simulink model "drone"  (Simulink 6.1)
settings: Solver=ode5  StartTime=0.0  StopTime=90  FixedStep=1e-2  RelTol=1e-3
undefined symbols (not defined in the file or in its folder): Aerodynamique, Correcteur, Mecanique
libraries: simulink x32, mblibv1 x29, aerolibtransform2 x4
(part 2 of 2)

== system drone/Electronique/Gestion Dynamique/Calcul Attitude/Norme ==
  Entrée : Inport  Port=1  LatchInput=off
  Add : Sum  Inputs=+++  OutScaling=2^-10
  Carré : simulink/Math Operations/Polynomial  coefs=[1 0 0]
  Carré1 : simulink/Math Operations/Polynomial  coefs=[1 0 0]
  Carré2 : simulink/Math Operations/Polynomial  coefs=[1 0 0]
  Demux2 : Demux  Outputs=3
  Math Function : Math  Operator=sqrt  SaturateOnIntegerOverflow=on
  Sortie : Outport
      settings: BusObject=perturbations
  wires:
  Math Function/1 -> Sortie/1
  Carré/1 -> Add/1
  Add/1 -> Math Function/1
  Carré1/1 -> Add/2
  Carré2/1 -> Add/3
  Demux2/2 -> Carré1/1
  Demux2/1 -> Carré/1
  Demux2/3 -> Carré2/1
  Entrée/1 -> Demux2/1

== system drone/Electronique/Gestion Dynamique/Calcul Attitude/Norme1 ==
  Entrée : Inport  Port=1  LatchInput=off
  Add : Sum  Inputs=+++  OutScaling=2^-10
  Carré : simulink/Math Operations/Polynomial  coefs=[1 0 0]
  Carré1 : simulink/Math Operations/Polynomial  coefs=[1 0 0]
  Carré2 : simulink/Math Operations/Polynomial  coefs=[1 0 0]
  Demux2 : Demux  Outputs=3
  Math Function : Math  Operator=sqrt  SaturateOnIntegerOverflow=on
  Sortie : Outport
      settings: BusObject=perturbations
  wires:
  Math Function/1 -> Sortie/1
  Carré/1 -> Add/1
  Add/1 -> Math Function/1
  Carré1/1 -> Add/2
  Carré2/1 -> Add/3
  Demux2/2 -> Carré1/1
  Demux2/1 -> Carré/1
  Demux2/3 -> Carré2/1
  Entrée/1 -> Demux2/1

== system drone/Electronique/Gestion Dynamique/Calcul Attitude/PID Attitude Ang ==
  Entrée : Inport  Port=1  LatchInput=off
  Derivative : Derivative
  Derivative2 : Derivative
  Gain : Gain  Gain=Correcteur.Attitude.Angle.Kp
  Gain1 : Gain  Gain=Correcteur.Attitude.Angle.Kd
  Gain2 : Gain  Gain=Correcteur.Attitude.Angle.Ki
  Gain3 : Gain  Gain=Correcteur.Attitude.Angle.Kdd
  Integrator : Integrator
  Reshape : simulink/Math Operations/Reshape  OutputDimensionality=1-D array  OutputDimensions=[1,1]
  Sum : Sum  Inputs=++++
  Sortie : Outport
      settings: BusObject=perturbations
  wires:
  Entrée/1 -> Gain/1
  Gain/1 -> Gain1/1, Gain2/1, Sum/3
  Gain2/1 -> Integrator/1
  Gain1/1 -> Derivative/1
  Sum/1 -> Reshape/1
  Reshape/1 -> Sortie/1
  Gain3/1 -> Derivative2/1
  Derivative2/1 -> Sum/1
  Integrator/1 -> Sum/4
  Derivative/1 -> Sum/2, Gain3/1

== system drone/Electronique/Gestion Dynamique/Calcul Attitude/PID Attitude Quat ==
  Entrée : Inport  Port=1  LatchInput=off
  Derivative : Derivative
  Derivative2 : Derivative
  Gain : Gain  Gain=Correcteur.Attitude.Quaternion.Kp
  Gain1 : Gain  Gain=Correcteur.Attitude.Quaternion.Kd
  Gain2 : Gain  Gain=Correcteur.Attitude.Quaternion.Ki
  Gain3 : Gain  Gain=Correcteur.Attitude.Quaternion.Kdd
  Integrator : Integrator
  Reshape : simulink/Math Operations/Reshape  OutputDimensionality=1-D array  OutputDimensions=[1,1]
  Sum : Sum  Inputs=++++
  Sortie : Outport
      settings: BusObject=perturbations
  wires:
  Entrée/1 -> Gain/1
  Gain/1 -> Gain1/1, Gain2/1, Sum/3
  Gain2/1 -> Integrator/1
  Gain1/1 -> Derivative/1
  Sum/1 -> Reshape/1
  Reshape/1 -> Sortie/1
  Gain3/1 -> Derivative2/1
  Derivative2/1 -> Sum/1
  Integrator/1 -> Sum/4
  Derivative/1 -> Sum/2, Gain3/1

== system drone/Electronique/Gestion Dynamique/Calcul Attitude/PID Attitude Vec ==
  Entrée : Inport  Port=1  LatchInput=off
  Derivative : Derivative
  Derivative2 : Derivative
  Gain : Gain  Gain=Correcteur.Attitude.Vecteur.Kp
  Gain1 : Gain  Gain=Correcteur.Attitude.Vecteur.Kd
  Gain2 : Gain  Gain=Correcteur.Attitude.Vecteur.Ki
  Gain3 : Gain  Gain=Correcteur.Attitude.Vecteur.Kdd
  Integrator : Integrator
  Reshape : simulink/Math Operations/Reshape  OutputDimensionality=1-D array  OutputDimensions=[1,1]
  Sum : Sum  Inputs=++++
  Sortie : Outport
      settings: BusObject=perturbations
  wires:
  Entrée/1 -> Gain/1
  Gain/1 -> Gain1/1, Gain2/1, Sum/3
  Gain2/1 -> Integrator/1
  Gain1/1 -> Derivative/1
  Sum/1 -> Reshape/1
  Reshape/1 -> Sortie/1
  Gain3/1 -> Derivative2/1
  Derivative2/1 -> Sum/1
  Integrator/1 -> Sum/4
  Derivative/1 -> Sum/2, Gain3/1

== system drone/Electronique/Gestion Dynamique/Calcul Attitude/inversion non infinie ==
  Entree : Inport  Port=1  LatchInput=off
  Constant : Constant
  Divide : Product  Inputs=/  OutScaling=2^-10
  Switch : Switch  Criteria=u2 > Threshold  ZeroCross=off
  Sortie : Outport
  wires:
  Switch/1 -> Divide/1
  Entree/1 -> Switch/1, Switch/2
  Constant/1 -> Switch/3
  Divide/1 -> Sortie/1

== system drone/Electronique/Gestion Dynamique/Calcul Position/Inverse quaternion ==
  Q : Inport  Port=1  LatchInput=off
  Gain : Gain  Gain=[1 -1 -1 -1]
  Q^-1 : Outport
  wires:
  Q/1 -> Gain/1
  Gain/1 -> Q^-1/1

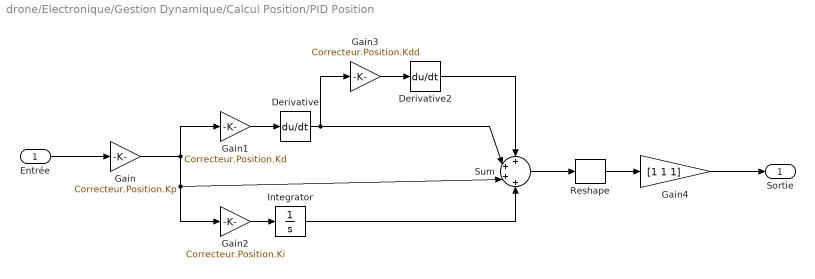
== system drone/Electronique/Gestion Dynamique/Calcul Position/PID Position ==
  Entrée : Inport  Port=1  LatchInput=off
  Derivative : Derivative
  Derivative2 : Derivative
  Gain : Gain  Gain=Correcteur.Position.Kp
  Gain1 : Gain  Gain=Correcteur.Position.Kd
  Gain2 : Gain  Gain=Correcteur.Position.Ki
  Gain3 : Gain  Gain=Correcteur.Position.Kdd
  Gain4 : Gain  Gain=[1 1 1]
  Integrator : Integrator
  Reshape : simulink/Math Operations/Reshape  OutputDimensionality=1-D array  OutputDimensions=[1,1]
  Sum : Sum  Inputs=++++
  Sortie : Outport
      settings: BusObject=perturbations
  wires:
  Entrée/1 -> Gain/1
  Gain/1 -> Gain1/1, Gain2/1, Sum/3
  Gain2/1 -> Integrator/1
  Gain1/1 -> Derivative/1
  Sum/1 -> Reshape/1
  Reshape/1 -> Gain4/1
  Gain3/1 -> Derivative2/1
  Derivative2/1 -> Sum/1
  Integrator/1 -> Sum/4
  Derivative/1 -> Sum/2, Gain3/1
  Gain4/1 -> Sortie/1

== system drone/Electronique/Gestion Dynamique/Separation composantes et erreur de position/Inverse quaternion ==
  Q : Inport  Port=1  LatchInput=off
  Gain : Gain  Gain=[1 -1 -1 -1]
  Q^-1 : Outport
  wires:
  Q/1 -> Gain/1
  Gain/1 -> Q^-1/1

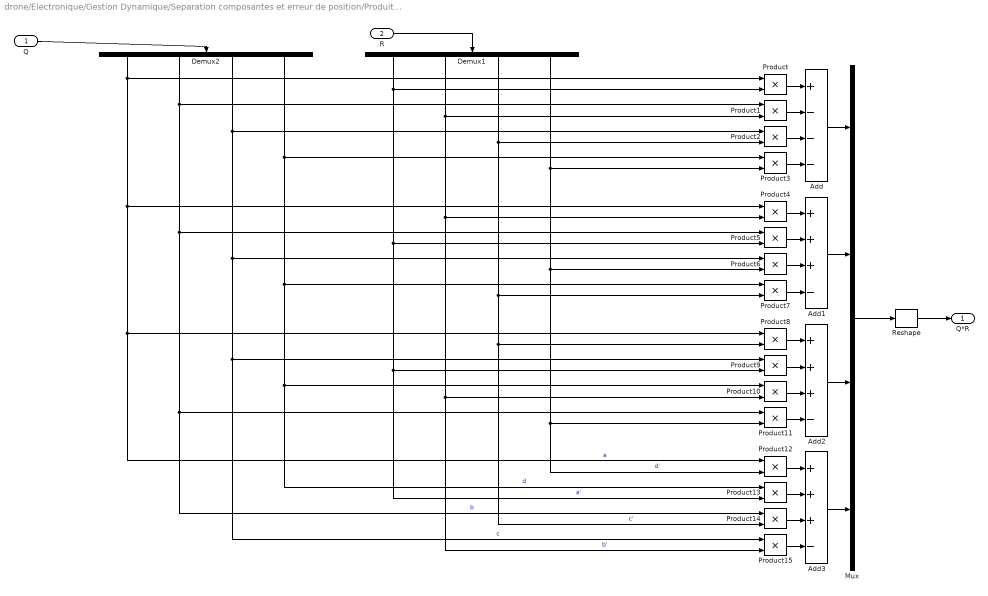
== system drone/Electronique/Gestion Dynamique/Separation composantes et erreur de position/Produit quaternion ==
  Q : Inport  Port=1  LatchInput=off
  R : Inport  Port=2  LatchInput=off
  Add : Sum  Inputs=+---  OutScaling=2^-10
  Add1 : Sum  Inputs=+++-  OutScaling=2^-10
  Add2 : Sum  Inputs=+++-  OutScaling=2^-10
  Add3 : Sum  Inputs=+++-  OutScaling=2^-10
  Demux1 : Demux  Orientation=down
  Demux2 : Demux  Orientation=down
  Mux : Mux
  Product{,1..15} (16 alike) : Product  RndMeth=Zero
  Reshape : simulink/Math Operations/Reshape  OutputDimensionality=1-D array  OutputDimensions=[1,1]
  Q*R : Outport
  wires:
  R/1 -> Demux1/1
  Q/1 -> Demux2/1
  Mux/1 -> Reshape/1
  Reshape/1 -> Q*R/1
  Demux2/1 -> Product/1, Product4/1, Product8/1, Product12/1  "a"
  Add/1 -> Mux/1
  Add1/1 -> Mux/2
  Add2/1 -> Mux/3
  Add3/1 -> Mux/4
  Product3/1 -> Add/4
  Product2/1 -> Add/3
  Product1/1 -> Add/2
  Product/1 -> Add/1
  Product7/1 -> Add1/4
  Product6/1 -> Add1/3
  Product5/1 -> Add1/2
  Product4/1 -> Add1/1
  Product11/1 -> Add2/4
  Product10/1 -> Add2/3
  Product9/1 -> Add2/2
  Product8/1 -> Add2/1
  Product15/1 -> Add3/4
  Product14/1 -> Add3/3
  Product13/1 -> Add3/2
  Product12/1 -> Add3/1
  Demux2/2 -> Product1/1, Product5/1, Product11/1, Product14/1  "b"
  Demux2/3 -> Product2/1, Product6/1, Product9/1, Product15/1  "c"
  Demux2/4 -> Product3/1, Product7/1, Product10/1, Product13/1  "d"
  Demux1/1 -> Product/2, Product5/2, Product9/2, Product13/2  "a'"
  Demux1/2 -> Product1/2, Product4/2, Product10/2, Product15/2  "b'"
  Demux1/3 -> Product2/2, Product7/2, Product8/2, Product14/2  "c'"
  Demux1/4 -> Product3/2, Product6/2, Product11/2, Product12/2  "d'"
